simulink model "Md61Md62CalibSet"  (R2018b)
settings: Solver=FixedStepDiscrete  StartTime=0.0  StopTime=10.0  FixedStep=0.01  RelTol=1e-3
undefined symbols (not defined in the file or in its folder): KeSMSuFirstRwStBackPosDelta_Val, KeSMSuFirstRwStCushFoldPosDelta_Val, KeSMSuFirstRwStFwdBkwdPosDelta_Val, KeSMSuThrdRwCushFoldPosDelta_Val, KeSMSwAcsMd30PassStBkReclnUpwdDnwdPos1_Val, KeSMSwAcsMd30PassStBkReclnUpwdDnwdPos1Max_Val, KeSMSwAcsMd30PassStBkReclnUpwdDnwdPos1Min_Val, KeSMSwAcsMd30PassStFldUpwdDnwdPos1_Val, KeSMSwAcsMd30PassStFrwdBkwdPos1_Val, KeSMSwAcsMd30PassStFrwdBkwdPos1Max_Val, KeSMSwAcsMd30PassStFrwdBkwdPos1Min_Val, KeSMSwSeatBkLimitPos_Val, KeSMSwSeatBkLimitPosDelt_Val
libraries: StIsPosChkLib x2
(part 4 of 5)

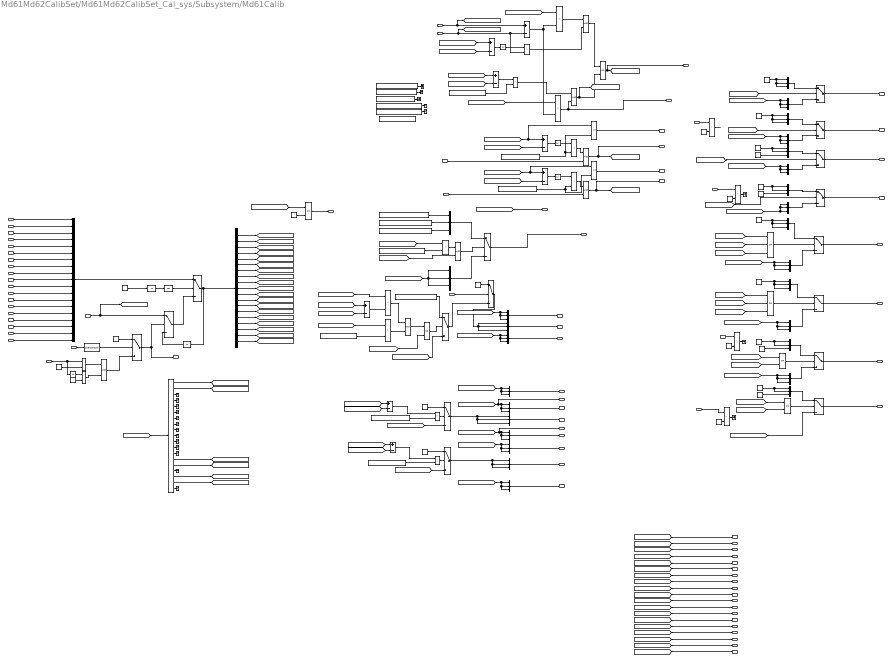
== system Md61Md62CalibSet/Md61Md62CalibSet_Cal_sys/Subsystem/Md61Calib ==
  EepMd61PassStBkReclnTrgtPos_Val_read : Inport
  EepMd61PassStCshnFldTrgtPos_Val_read : Inport  Port=2
  EepMd61PassStFwdBkwdTrgtPos_Val_read : Inport  Port=3
  EepMd61SecRwLtStBkReclnTrgtPos_Val_read : Inport  Port=4
  EepMd61SecRwLtStCushFrntTrgtPos_Val_read : Inport  Port=5
  EepMd61SecRwLtStFwdBkwdTrgtPos_Val_read : Inport  Port=6
  EepMd61SecRwLtStLgrstInwdOtwdTrgtPos_Val_read : Inport  Port=7
  EepMd61SecRwLtStLgrstUpwdDnwdTrgtPos_Val_read : Inport  Port=8
  EepMd61SecRwRtStBkReclnTrgtPos_Val_read : Inport  Port=9
  EepMd61SecRwRtStCushFrntTrgtPos_Val_read : Inport  Port=10
  EepMd61SecRwRtStFwdBkwdTrgtPos_Val_read : Inport  Port=11
  EepMd61SecRwRtStLgrstInwdOtwdTrgtPos_Val_read : Inport  Port=12
  EepMd61SecRwRtStLgrstUpwdDnwdTrgtPos_Val_read : Inport  Port=13
  EepMd61ThdRwLtStBkReclnTrgtPos_Val_read : Inport  Port=14
  EepMd61ThdRwLtStCshnFldTrgtPos_Val_read : Inport  Port=15
  EepMd61ThdRwLtStFwdBkwdTrgtPos_Val_read : Inport  Port=16
  EepMd61ThdRwRtStBkReclnTrgtPos_Val_read : Inport  Port=17
  EepMd61ThdRwRtStCshnFldTrgtPos_Val_read : Inport  Port=18
  EepMd61ThdRwRtStFwdBkwdTrgtPos_Val_read : Inport  Port=19
  CurrentPosArray : Inport  Port=20
  MemReq : Inport  Port=21
  ThdRwLtStCshnFldUpwdDnwdMovConfig : Inport  Port=22
  ThdRwRtStCshnFldUpwdDnwdMovConfig : Inport  Port=23
  KeSMSwSeatBkLimitPos_Val : Inport  Port=24
  KeSMSwSeatBkLimitPosDelt_Val : Inport  Port=25
  IfVeSMSuPassStBkReclnUpwdDnwdPosV_Val_read : Inport  Port=26
  IfVeSMSuSecRwRtStBkReclnUpwdDnwdPos : Inport  Port=27
  IfVeSMSuSecRwLtStFrwdBkwdPos : Inport  Port=28
  IfVeSMSuSecRwLtStBkReclnUpwdDnwdPos : Inport  Port=29
  IfVeSMSuSecRwRtStFrwdBkwdPos : Inport  Port=30
  modestate32_Val_read : Inport  Port=31
  32BitSelector1 : StIsPosChkLib/32BitSelector  BitNum=5
  Abs : Abs
  Abs1 : Abs
  Abs2 : Abs
  Add{,1..3,6..7} (6 alike) : Sum  Inputs=+-  OutDataTypeStr=int16
  Add4 : Sum  Inputs=+-  AccumDataTypeStr=int16  OutDataTypeStr=int16
  Add5 : Sum  Inputs=+-  AccumDataTypeStr=int16  OutDataTypeStr=int16
  Constant : Constant  Value=0  OutDataTypeStr=boolean
  Constant1 : Constant  Value=4  OutDataTypeStr=uint8
  Constant{5..6,9..11,14,26..27} (8 alike) : Constant  Value=0  OutDataTypeStr=uint16
  Constant{7,12,22,24} (4 alike) : Constant  Value=1280  OutDataTypeStr=uint16
  Constant{8,13,23,25} (4 alike) : Constant  Value=480  OutDataTypeStr=uint16
  Constant16 : Constant  Value=4000  OutDataTypeStr=uint16
  Constant18 : Constant  Value=4000  OutDataTypeStr=uint16
  Constant2 : Constant  Value=4  OutDataTypeStr=uint8
  Constant20 : Constant  Value=4095  OutDataTypeStr=uint16
  Constant3 : Constant  Value=0  OutDataTypeStr=uint8
  Constant4 : Constant  Value=4095
  Demux : Demux  Outputs=19
  Demux1 : Demux  Outputs=19
  Logical Operator{,1..3,5,10..11} (7 alike) : Logic  AllPortsSameDT=off  OutDataTypeStr=boolean
  Logical Operator{4,8..9,12} (4 alike) : Logic  Operator=OR  AllPortsSameDT=off  OutDataTypeStr=boolean
  Logical Operator6 : Logic  Operator=OR  Inputs=3  AllPortsSameDT=off  OutDataTypeStr=boolean
  Logical Operator7 : Logic  Operator=OR  Inputs=3  AllPortsSameDT=off  OutDataTypeStr=boolean
  Mux : Mux  Inputs=19
  Mux{2..28} (27 alike) : Mux  Inputs=3
  PA_KeSMSuFirstRwStBackPosDelta_Val : Constant  Value=KeSMSuFirstRwStBackPosDelta_Val
  PA_KeSMSuFirstRwStBackPosDelta_Val1 : Constant  Value=KeSMSuFirstRwStBackPosDelta_Val
  PA_KeSMSuFirstRwStBackPosDelta_Val2 : Constant  Value=KeSMSuFirstRwStBackPosDelta_Val
  PA_KeSMSuFirstRwStCushFoldPosDelta_Val : Constant  Value=KeSMSuFirstRwStCushFoldPosDelta_Val
  PA_KeSMSuFirstRwStFwdBkwdPosDelta_Val : Constant  Value=KeSMSuFirstRwStFwdBkwdPosDelta_Val
  PA_KeSMSuThrdRwCushFoldPosDelta_Val{,1..4} (5 alike) : Constant  Value=KeSMSuThrdRwCushFoldPosDelta_Val
  PA_KeSMSwAcsMd30PassStBkReclnUpwdDnwdPos1Max_Val1 : Constant  Value=KeSMSwAcsMd30PassStBkReclnUpwdDnwdPos1Max_Val
  PA_KeSMSwAcsMd30PassStBkReclnUpwdDnwdPos1Min_Val1 : Constant  Value=KeSMSwAcsMd30PassStBkReclnUpwdDnwdPos1Min_Val
  PA_KeSMSwAcsMd30PassStBkReclnUpwdDnwdPos1_Val1 : Constant  Value=KeSMSwAcsMd30PassStBkReclnUpwdDnwdPos1_Val
  PA_KeSMSwAcsMd30PassStFldUpwdDnwdPos1_Val : Constant  Value=KeSMSwAcsMd30PassStFldUpwdDnwdPos1_Val
  PA_KeSMSwAcsMd30PassStFrwdBkwdPos1Max_Val : Constant  Value=KeSMSwAcsMd30PassStFrwdBkwdPos1Max_Val
  PA_KeSMSwAcsMd30PassStFrwdBkwdPos1Min_Val : Constant  Value=KeSMSwAcsMd30PassStFrwdBkwdPos1Min_Val
  PA_KeSMSwAcsMd30PassStFrwdBkwdPos1_Val : Constant  Value=KeSMSwAcsMd30PassStFrwdBkwdPos1_Val
  Relational Operator : RelationalOperator  Operator===  OutDataTypeStr=boolean  RndMeth=Simplest
  Relational Operator1 : RelationalOperator  Operator=~=  OutDataTypeStr=boolean  RndMeth=Simplest
  Relational Operator10 : RelationalOperator  Operator=<=  OutDataTypeStr=boolean  RndMeth=Simplest
  Relational Operator{2..3,8,11..12,14..20} (12 alike) : RelationalOperator  Operator=>  OutDataTypeStr=boolean  RndMeth=Simplest
  Relational Operator13 : RelationalOperator  Operator=<  OutDataTypeStr=boolean  RndMeth=Simplest
  Relational Operator4 : RelationalOperator  Operator=<  OutDataTypeStr=boolean  RndMeth=Simplest
  Relational Operator6 : RelationalOperator  Operator=<  OutDataTypeStr=boolean  RndMeth=Simplest
  Relational Operator7 : RelationalOperator  Operator===  OutDataTypeStr=boolean  RndMeth=Simplest
  Relational Operator9 : RelationalOperator  Operator=<=  OutDataTypeStr=boolean  RndMeth=Simplest
  Switch{,1..15} (16 alike) : Switch  Criteria=u2 > Threshold
  Terminator_{2..22} (21 alike) : Terminator
  Unit Delay : UnitDelay  InitialCondition=1  SampleTime=-1
  Unit Delay1 : UnitDelay  InitialCondition=1  SampleTime=-1
  Unit Delay2 : UnitDelay  InitialCondition=1  SampleTime=-1
  Unit Delay3 : UnitDelay  SampleTime=-1
  Md61PassStBkReclnTrgtPos_Val_write : Outport
      settings: EnsureOutportIsVirtual=on
  Md61PassStBkReclnTrgtPosCalib_TrgtPosArray_write : Outport  Port=2
      settings: EnsureOutportIsVirtual=on
  Md61PassStCshnFldTrgtPosCalib_TrgtPosArray_write : Outport  Port=3
      settings: EnsureOutportIsVirtual=on
  Md61PassStFwdBkwdTrgtPosCalib_TrgtPosArray_write : Outport  Port=4
      settings: EnsureOutportIsVirtual=on
  Md61SecRwLtStBkReclnTrgtPosCalib_TrgtPosArray_write : Outport  Port=5
      settings: EnsureOutportIsVirtual=on
  Md61SecRwLtStCushFrntTrgtPosCalib_TrgtPosArray_write : Outport  Port=6
      settings: EnsureOutportIsVirtual=on
  Md61SecRwLtStFwdBkwdCalib_TrgtPosArray_write : Outport  Port=7
      settings: EnsureOutportIsVirtual=on
  Md61SecRwLtStLgrstInwdOtwdTrgtPosCalib_TrgtPosArray_write : Outport  Port=8
      settings: EnsureOutportIsVirtual=on
  Md61SecRwLtStLgrstUpwdDnwdTrgtPosCalib_TrgtPosArray_write : Outport  Port=9
      settings: EnsureOutportIsVirtual=on
  Md61ThdRwLtStBkReclnUpwdDnwdTrgtPosCalib_TrgtPosArray_write : Outport  Port=10
      settings: EnsureOutportIsVirtual=on
  Md61ThdRwLtStCshnFldUpwdDnwdTrgtPos_Val_write : Outport  Port=11
      settings: EnsureOutportIsVirtual=on
  Md61ThdRwLtStCshnFldUpwdDnwdTrgtPosCalib_TrgtPosArray_write : Outport  Port=12
      settings: EnsureOutportIsVirtual=on
  Md61ThdRwLtStFrwdBkwdPosTrgtPosCalib_TrgtPosArray_write : Outport  Port=13
      settings: EnsureOutportIsVirtual=on
  Md61ThdRwRtStCshnFldUpwdDnwdTrgtPos_Val_write : Outport  Port=14
      settings: EnsureOutportIsVirtual=on
  Md61SecRwRtStBkReclnTrgtPosCalib_TrgtPosArray_write : Outport  Port=15
      settings: EnsureOutportIsVirtual=on
  Md61SecRwRtStCushFrntTrgtPosCalib_TrgtPosArray_write : Outport  Port=16
      settings: EnsureOutportIsVirtual=on
  Md61SecRwRtStFwdBkwdCalib_TrgtPosArray_write : Outport  Port=17
      settings: EnsureOutportIsVirtual=on
  Md61SecRwRtStLgrstInwdOtwdTrgtPosCalib_TrgtPosArray_write : Outport  Port=18
      settings: EnsureOutportIsVirtual=on
  Md61SecRwRtStLgrstUpwdDnwdTrgtPosCalib_TrgtPosArray_write : Outport  Port=19
      settings: EnsureOutportIsVirtual=on
  Md61ThdRwRtStBkReclnUpwdDnwdTrgtPosCalib_TrgtPosArray_write : Outport  Port=20
      settings: EnsureOutportIsVirtual=on
  Md61ThdRwRtStCshnFldUpwdDnwdTrgtPosCalib_TrgtPosArray_write : Outport  Port=21
      settings: EnsureOutportIsVirtual=on
  Md61ThdRwRtStFrwdBkwdPosTrgtPosCalib_TrgtPosArray_write : Outport  Port=22
      settings: EnsureOutportIsVirtual=on
  Md61PassStNeedFldOpn_Val_write : Outport  Port=23
      settings: EnsureOutportIsVirtual=on
  Md61PassStTrgtIsFld_Val_write : Outport  Port=24
      settings: EnsureOutportIsVirtual=on
  Md61ThdRwLtStNeedFldOpn_Val_write : Outport  Port=25
      settings: EnsureOutportIsVirtual=on
  Md61ThdRwLtStTrgtIsFld_Val_write : Outport  Port=26
      settings: EnsureOutportIsVirtual=on
  Md61ThdRwRtStNeedFldOpn_Val_write : Outport  Port=27
      settings: EnsureOutportIsVirtual=on
  Md61ThdRwRtStTrgtIsFld_Val_write : Outport  Port=28
      settings: EnsureOutportIsVirtual=on
  EepMd61PassStBkReclnTrgtPos_S_Val_write : Outport  Port=29
      settings: EnsureOutportIsVirtual=on
  EepMd61PassStCshnFldTrgtPos_S_Val_write : Outport  Port=30
      settings: EnsureOutportIsVirtual=on
  EepMd61PassStFwdBkwdTrgtPos_S_Val_write : Outport  Port=31
      settings: EnsureOutportIsVirtual=on
  EepMd61SecRwLtStBkReclnTrgtPos_S_Val_write : Outport  Port=32
      settings: EnsureOutportIsVirtual=on
  EepMd61SecRwLtStCushFrntTrgtPos_S_Val_write : Outport  Port=33
      settings: EnsureOutportIsVirtual=on
  EepMd61SecRwLtStFwdBkwdTrgtPos_S_Val_write : Outport  Port=34
      settings: EnsureOutportIsVirtual=on
  EepMd61SecRwLtStLgrstInwdOtwdTrgtPos_S_Val_write : Outport  Port=35
      settings: EnsureOutportIsVirtual=on
  EepMd61SecRwLtStLgrstUpwdDnwdTrgtPos_S_Val_write : Outport  Port=36
      settings: EnsureOutportIsVirtual=on
  EepMd61SecRwRtStBkReclnTrgtPos_S_Val_write : Outport  Port=37
      settings: EnsureOutportIsVirtual=on
  EepMd61SecRwRtStCushFrntTrgtPos_S_Val_write : Outport  Port=38
      settings: EnsureOutportIsVirtual=on
  EepMd61SecRwRtStFwdBkwdTrgtPos_S_Val_write : Outport  Port=39
      settings: EnsureOutportIsVirtual=on
  EepMd61SecRwRtStLgrstInwdOtwdTrgtPos_S_Val_write : Outport  Port=40
      settings: EnsureOutportIsVirtual=on
  EepMd61SecRwRtStLgrstUpwdDnwdTrgtPos_S_Val_write : Outport  Port=41
      settings: EnsureOutportIsVirtual=on
  EepMd61ThdRwLtStBkReclnTrgtPos_S_Val_write : Outport  Port=42
      settings: EnsureOutportIsVirtual=on
  EepMd61ThdRwLtStCshnFldTrgtPos_S_Val_write : Outport  Port=43
      settings: EnsureOutportIsVirtual=on
  EepMd61ThdRwLtStFwdBkwdTrgtPos_S_Val_write : Outport  Port=44
      settings: EnsureOutportIsVirtual=on
  EepMd61ThdRwRtStBkReclnTrgtPos_S_Val_write : Outport  Port=45
      settings: EnsureOutportIsVirtual=on
  EepMd61ThdRwRtStCshnFldTrgtPos_S_Val_write : Outport  Port=46
      settings: EnsureOutportIsVirtual=on
  EepMd61ThdRwRtStFwdBkwdTrgtPos_S_Val_write : Outport  Port=47
      settings: EnsureOutportIsVirtual=on
  Md61MemReq_Val_write : Outport  Port=48
      settings: EnsureOutportIsVirtual=on
  Md61NotMem_Val_write : Outport  Port=49
      settings: EnsureOutportIsVirtual=on
  wires:
  Unit Delay/1 -> Unit Delay1/1
  Constant/1 -> Unit Delay/1
  Unit Delay1/1 -> Switch/2
  Switch1/1 -> Switch/3
  EepMd61ThdRwRtStFwdBkwdTrgtPos_Val_read/1 -> Mux/19
  EepMd61ThdRwRtStCshnFldTrgtPos_Val_read/1 -> Mux/18
  EepMd61ThdRwRtStBkReclnTrgtPos_Val_read/1 -> Mux/17
  EepMd61ThdRwLtStFwdBkwdTrgtPos_Val_read/1 -> Mux/16
  EepMd61ThdRwLtStCshnFldTrgtPos_Val_read/1 -> Mux/15
  EepMd61ThdRwLtStBkReclnTrgtPos_Val_read/1 -> Mux/14
  EepMd61SecRwRtStLgrstUpwdDnwdTrgtPos_Val_read/1 -> Mux/13
  EepMd61SecRwRtStLgrstInwdOtwdTrgtPos_Val_read/1 -> Mux/12
  EepMd61SecRwRtStFwdBkwdTrgtPos_Val_read/1 -> Mux/11
  EepMd61SecRwRtStCushFrntTrgtPos_Val_read/1 -> Mux/10
  EepMd61SecRwRtStBkReclnTrgtPos_Val_read/1 -> Mux/9
  EepMd61SecRwLtStLgrstUpwdDnwdTrgtPos_Val_read/1 -> Mux/8
  EepMd61SecRwLtStLgrstInwdOtwdTrgtPos_Val_read/1 -> Mux/7
  EepMd61SecRwLtStFwdBkwdTrgtPos_Val_read/1 -> Mux/6
  EepMd61SecRwLtStCushFrntTrgtPos_Val_read/1 -> Mux/5
  EepMd61SecRwLtStBkReclnTrgtPos_Val_read/1 -> Mux/4
  EepMd61PassStFwdBkwdTrgtPos_Val_read/1 -> Mux/3
  EepMd61PassStCshnFldTrgtPos_Val_read/1 -> Mux/2
  EepMd61PassStBkReclnTrgtPos_Val_read/1 -> Mux/1
  Mux/1 -> Switch/1
  CurrentPosArray/1 -> [CurrentPosArray], Switch1/1
  Unit Delay2/1 -> Switch1/3
  MemReq/1 -> Unit Delay3/1, Relational Operator/1
  Constant1/1 -> Relational Operator/2
  Relational Operator/1 -> Logical Operator/1
  Unit Delay3/1 -> Relational Operator1/1
  Constant2/1 -> Relational Operator1/2
  Relational Operator1/1 -> Logical Operator/2
  Demux/15 -> [ThdRwLtStCshnFldTrgtPos]
  Demux/16 -> [ThdRwLtStFwdBkwdTrgtPos]
  Demux/5 -> [SecRwLtStCushFrntTrgtPos]
  Demux/17 -> [ThdRwRtStBkReclnTrgtPos]
  Demux/14 -> [ThdRwLtStBkReclnTrgtPos]
  Demux/9 -> [SecRwRtStBkReclnTrgtPos]
  Demux/13 -> [SecRwRtStLgrstUpwdDnwdTrgtPos]
  Demux/19 -> [ThdRwRtStFwdBkwdTrgtPos]
  Demux/11 -> [SecRwRtStFwdBkwdTrgtPos]
  Switch/1 -> Demux/1, Unit Delay2/1
  Demux/8 -> [SecRwLtStLgrstUpwdDnwdTrgtPos]
  Demux/2 -> [PassStCshnFldTrgtPos]
  Demux/12 -> [SecRwRtStLgrstInwdOtwdTrgtPos]
  Demux/7 -> [SecRwLtStLgrstInwdOtwdTrgtPos]
  Demux/6 -> [SecRwLtStFwdBkwdTrgtPos]
  Demux/4 -> [SecRwLtStBkReclnTrgtPos]
  Demux/3 -> [PassStFwdBkwdTrgtPos]
  Demux/1 -> [PassStBkReclnTrgtPos]
  Demux/10 -> [SecRwRtStCushFrntTrgtPos]
  Demux/18 -> [ThdRwRtStCshnFldTrgtPos]
  Mux2/1 -> Md61PassStCshnFldTrgtPosCalib_TrgtPosArray_write/1
  [PassStCshnFldTrgtPos] -> Mux2/1, Mux2/2, Mux2/3
  Mux3/1 -> Md61PassStFwdBkwdTrgtPosCalib_TrgtPosArray_write/1
  Mux4/1 -> Md61SecRwLtStCushFrntTrgtPosCalib_TrgtPosArray_write/1
  [SecRwLtStCushFrntTrgtPos] -> Mux4/1, Mux4/2, Mux4/3
  [ThdRwLtStBkReclnTrgtPos] -> Mux5/3, Mux5/2, Mux5/1
  Mux5/1 -> Md61ThdRwLtStBkReclnUpwdDnwdTrgtPosCalib_TrgtPosArray_write/1
  [ThdRwLtStCshnFldTrgtPos] -> Md61ThdRwLtStCshnFldUpwdDnwdTrgtPos_Val_write/1, Mux6/1, Mux6/2, Mux6/3
  Mux6/1 -> Md61ThdRwLtStCshnFldUpwdDnwdTrgtPosCalib_TrgtPosArray_write/1
  Mux7/1 -> Md61ThdRwLtStFrwdBkwdPosTrgtPosCalib_TrgtPosArray_write/1
  [ThdRwRtStCshnFldTrgtPos] -> Md61ThdRwRtStCshnFldUpwdDnwdTrgtPos_Val_write/1, Mux8/1, Mux8/2, Mux8/3
  [SecRwRtStCushFrntTrgtPos] -> Mux9/3, Mux9/2, Mux9/1
  Mux9/1 -> Md61SecRwRtStCushFrntTrgtPosCalib_TrgtPosArray_write/1
  Mux8/1 -> Md61ThdRwRtStCshnFldUpwdDnwdTrgtPosCalib_TrgtPosArray_write/1
  Mux10/1 -> Md61ThdRwRtStBkReclnUpwdDnwdTrgtPosCalib_TrgtPosArray_write/1
  [ThdRwRtStBkReclnTrgtPos] -> Mux10/3, Mux10/2, Mux10/1
  Mux11/1 -> Md61ThdRwRtStFrwdBkwdPosTrgtPosCalib_TrgtPosArray_write/1
  [CurrentPosArray] -> Demux1/1
  Demux1/17 -> [ThdRwRtStBkReclnPos]
  Demux1/14 -> [ThdRwLtStBkReclnPos]
  Demux1/18 -> [ThdRwRtStCshnFldPos]
  Demux1/1 -> [PassStBkReclnPos]
  Demux1/15 -> [ThdRwLtStCshnFldPos]
  Demux1/2 -> [PassStCshnFldPos]
  [ThdRwLtStCshnFldPos] -> Add/2
  Add/1 -> Abs/1
  Abs/1 -> Relational Operator2/1
  PA_KeSMSuThrdRwCushFoldPosDelta_Val1/1 -> Relational Operator9/2, Relational Operator2/2
  ThdRwLtStCshnFldUpwdDnwdMovConfig/1 -> Logical Operator1/2
  Relational Operator2/1 -> Logical Operator1/1
  Logical Operator1/1 -> Md61ThdRwLtStNeedFldOpn_Val_write/1, [ThdLftNeedFldOpn]
  ThdRwRtStCshnFldUpwdDnwdMovConfig/1 -> Logical Operator2/2
  Relational Operator3/1 -> Logical Operator2/1
  PA_KeSMSuThrdRwCushFoldPosDelta_Val2/1 -> Relational Operator3/2, Relational Operator10/2
  Abs1/1 -> Relational Operator3/1
  Add1/1 -> Abs1/1
  [ThdRwRtStCshnFldPos] -> Add1/2
  [ThdRwRtStCshnFldTrgtPos] -> Relational Operator10/1, Add1/1
  Logical Operator2/1 -> Md61ThdRwRtStNeedFldOpn_Val_write/1, [ThdRghtNeedFldOpn]
  Demux1/3 -> Terminator_2/1
  Demux1/4 -> Terminator_3/1
  Demux1/5 -> Terminator_4/1
  Demux1/6 -> Terminator_5/1
  Demux1/7 -> Terminator_6/1
  Demux1/8 -> Terminator_7/1
  Demux1/9 -> Terminator_8/1
  Demux1/10 -> Terminator_9/1
  Demux1/11 -> Terminator_10/1
  Demux1/12 -> Terminator_11/1
  Demux1/13 -> Terminator_12/1
  Demux1/16 -> Terminator_13/1
  Demux1/19 -> Terminator_14/1
  [ThdLftNeedFldOpn] -> Switch2/2
  Switch8/1 -> Md61SecRwRtStBkReclnTrgtPosCalib_TrgtPosArray_write/1
  KeSMSwSeatBkLimitPosDelt_Val/1 -> [SeatBkLimitPosDelt], Relational Operator8/2, Add2/2
  [PassStBkReclnPos] -> Relational Operator4/1
  Relational Operator4/1 -> Logical Operator3/1
  Logical Operator3/1 -> Logical Operator4/1
  Logical Operator4/1 -> Md61PassStNeedFldOpn_Val_write/1, [PassStNeedFldOpn]
  KeSMSwSeatBkLimitPos_Val/1 -> [SeatBkLimitPos], Add2/1
  Logical Operator5/1 -> [PassStNeedFld], Logical Operator4/2
  Relational Operator6/1 -> Md61PassStTrgtIsFld_Val_write/1, Logical Operator5/2
  Add2/1 -> Relational Operator6/2, Relational Operator4/2
  [PassStBkReclnTrgtPos] -> Relational Operator6/1
  [PassStBkReclnPos] -> Add3/2
  [PassStBkReclnTrgtPos] -> Add3/1
  Add3/1 -> Abs2/1
  Abs2/1 -> Relational Operator8/1
  Relational Operator8/1 -> Logical Operator3/2
  [ThdLftNeedFldOpn] -> Logical Operator6/1
  [ThdRghtNeedFldOpn] -> Logical Operator6/2
  Mux12/1 -> Switch2/1
  Switch2/1 -> Md61SecRwLtStLgrstInwdOtwdTrgtPosCalib_TrgtPosArray_write/1
  Switch3/1 -> Md61SecRwLtStLgrstUpwdDnwdTrgtPosCalib_TrgtPosArray_write/1
  [ThdLftNeedFldOpn] -> Switch3/2
  [SecRwLtStLgrstInwdOtwdTrgtPos] -> Mux13/1, Mux13/2, Mux13/3
  Mux13/1 -> Switch2/3
  Mux14/1 -> Switch3/3
  [SecRwLtStLgrstUpwdDnwdTrgtPos] -> Mux14/3, Mux14/2, Mux14/1
  Constant5/1 -> Mux12/3, Mux12/2, Mux12/1
  Constant6/1 -> Mux15/3, Mux15/2, Mux15/1
  Mux15/1 -> Switch3/1
  Switch4/1 -> Md61SecRwLtStBkReclnTrgtPosCalib_TrgtPosArray_write/1
  Switch5/1 -> Md61SecRwLtStFwdBkwdCalib_TrgtPosArray_write/1
  [SecRwLtStBkReclnTrgtPos] -> Mux16/1, Mux16/2, Mux16/3
  Mux16/1 -> Switch4/3
  Mux17/1 -> Switch5/3
  [SecRwLtStFwdBkwdTrgtPos] -> Mux17/1, Mux17/2, Mux17/3
  Mux18/1 -> Switch4/1
  Constant7/1 -> Mux18/1, Mux18/2
  Constant8/1 -> Mux19/2, Mux19/1
  Mux19/1 -> Switch5/1
  Constant9/1 -> Mux19/3
  [PassStNeedFldOpn] -> Logical Operator6/3
  Switch6/1 -> Md61SecRwRtStLgrstInwdOtwdTrgtPosCalib_TrgtPosArray_write/1
  Mux20/1 -> Switch6/1
  Logical Operator6/1 -> Switch6/2
  Logical Operator7/1 -> Switch7/2
  Mux21/1 -> Switch7/1
  Switch7/1 -> Md61SecRwRtStLgrstUpwdDnwdTrgtPosCalib_TrgtPosArray_write/1
  [PassStNeedFldOpn] -> Logical Operator7/3
  [ThdRghtNeedFldOpn] -> Logical Operator7/2
  [ThdLftNeedFldOpn] -> Logical Operator7/1
  Constant10/1 -> Mux20/1, Mux20/2, Mux20/3
  Constant11/1 -> Mux21/3, Mux21/2, Mux21/1
  [SecRwRtStLgrstInwdOtwdTrgtPos] -> Mux22/3, Mux22/2, Mux22/1
  Mux22/1 -> Switch6/3
  Mux23/1 -> Switch7/3
  [SecRwRtStLgrstUpwdDnwdTrgtPos] -> Mux23/3, Mux23/2, Mux23/1
  Switch9/1 -> Md61SecRwRtStFwdBkwdCalib_TrgtPosArray_write/1
  Mux24/1 -> Switch8/1
  [ThdLftNeedFldOpn] -> Logical Operator8/1
  [ThdRghtNeedFldOpn] -> Logical Operator8/2
  Constant12/1 -> Mux24/2, Mux24/1
  [SecRwRtStBkReclnTrgtPos] -> Mux25/1, Mux25/2, Mux25/3
  Mux25/1 -> Switch8/3
  Constant14/1 -> Mux26/3
  Mux26/1 -> Switch9/1
  Constant13/1 -> Mux26/1, Mux26/2
  [ThdRghtNeedFldOpn] -> Logical Operator9/2
  [ThdLftNeedFldOpn] -> Logical Operator9/1
  [SecRwRtStFwdBkwdTrgtPos] -> Switch9/3
  [ThdRwLtStCshnFldTrgtPos] -> Relational Operator9/1, Add/1
  Relational Operator10/1 -> Md61ThdRwRtStTrgtIsFld_Val_write/1
  Relational Operator9/1 -> Md61ThdRwLtStTrgtIsFld_Val_write/1
  [ThdRwLtStFwdBkwdTrgtPos] -> Switch10/3
  Switch10/1 -> Mux7/3, Mux7/2, Mux7/1
  [ThdRwLtStCshnFldTrgtPos] -> Add4/2
  [ThdRwLtStCshnFldPos] -> Add4/1
  Add4/1 -> Relational Operator11/1
  PA_KeSMSuThrdRwCushFoldPosDelta_Val3/1 -> Relational Operator11/2
  Relational Operator11/1 -> Switch10/2
  Constant16/1 -> Switch10/1
  Switch11/1 -> Mux11/3, Mux11/2, Mux11/1
  [ThdRwRtStFwdBkwdTrgtPos] -> Switch11/3
  Constant18/1 -> Switch11/1
  Add5/1 -> Relational Operator12/1
  Relational Operator12/1 -> Switch11/2
  [ThdRwRtStCshnFldTrgtPos] -> Add5/2
  PA_KeSMSuThrdRwCushFoldPosDelta_Val4/1 -> Relational Operator12/2
  [ThdRwRtStCshnFldPos] -> Add5/1
  [SeatBkLimitPos] -> Add6/1
  [SeatBkLimitPosDelt] -> Add6/2
  [PassStBkReclnPos] -> Relational Operator13/1
  Add6/1 -> Relational Operator13/2
  PA_KeSMSuFirstRwStBackPosDelta_Val1/1 -> Relational Operator14/2
  [PassStBkReclnPos] -> Relational Operator14/1
  Relational Operator13/1 -> Logical Operator10/1
  Relational Operator14/1 -> Logical Operator10/2
  [PassStFwdBkwdTrgtPos] -> Switch12/3
  Switch15/1 -> Mux3/2, Mux3/3, Mux3/1
  PA_KeSMSwAcsMd30PassStFrwdBkwdPos1_Val/1 -> Switch12/1
  PA_KeSMSwAcsMd30PassStFldUpwdDnwdPos1_Val/1 -> Relational Operator15/2
  [PassStCshnFldPos] -> Relational Operator15/1
  PA_KeSMSwAcsMd30PassStBkReclnUpwdDnwdPos1_Val1/1 -> Mux27/1
  PA_KeSMSwAcsMd30PassStBkReclnUpwdDnwdPos1Max_Val1/1 -> Mux27/2
  Mux27/1 -> Switch13/1
  [PassStBkReclnTrgtPos] -> Md61PassStBkReclnTrgtPos_Val_write/1
  [PassStBkReclnTrgtPos] -> Mux28/3, Mux28/1, Mux28/2
  Mux28/1 -> Switch13/3
  Switch13/1 -> Md61PassStBkReclnTrgtPosCalib_TrgtPosArray_write/1
  Relational Operator15/1 -> Logical Operator11/1
  Logical Operator11/1 -> Switch13/2
  [PassStBkReclnPos] -> Add7/1
  [PassStBkReclnTrgtPos] -> Add7/2
  Add7/1 -> Relational Operator16/1
  PA_KeSMSuFirstRwStBackPosDelta_Val/1 -> Relational Operator16/2
  Relational Operator16/1 -> Logical Operator5/1
  [PassStNeedFld] -> Logical Operator11/2
  PA_KeSMSwAcsMd30PassStBkReclnUpwdDnwdPos1Min_Val1/1 -> Mux27/3
  [PassStBkReclnTrgtPos] -> EepMd61PassStBkReclnTrgtPos_S_Val_write/1
  [PassStCshnFldTrgtPos] -> EepMd61PassStCshnFldTrgtPos_S_Val_write/1
  [PassStFwdBkwdTrgtPos] -> EepMd61PassStFwdBkwdTrgtPos_S_Val_write/1
  [SecRwLtStBkReclnTrgtPos] -> EepMd61SecRwLtStBkReclnTrgtPos_S_Val_write/1
  [SecRwLtStCushFrntTrgtPos] -> EepMd61SecRwLtStCushFrntTrgtPos_S_Val_write/1
  [ThdRwRtStFwdBkwdTrgtPos] -> EepMd61ThdRwRtStFwdBkwdTrgtPos_S_Val_write/1
  [ThdRwRtStCshnFldTrgtPos] -> EepMd61ThdRwRtStCshnFldTrgtPos_S_Val_write/1
  [ThdRwRtStBkReclnTrgtPos] -> EepMd61ThdRwRtStBkReclnTrgtPos_S_Val_write/1
  [ThdRwLtStFwdBkwdTrgtPos] -> EepMd61ThdRwLtStFwdBkwdTrgtPos_S_Val_write/1
  [ThdRwLtStCshnFldTrgtPos] -> EepMd61ThdRwLtStCshnFldTrgtPos_S_Val_write/1
  [ThdRwLtStBkReclnTrgtPos] -> EepMd61ThdRwLtStBkReclnTrgtPos_S_Val_write/1
  [SecRwRtStLgrstUpwdDnwdTrgtPos] -> EepMd61SecRwRtStLgrstUpwdDnwdTrgtPos_S_Val_write/1
  [SecRwRtStLgrstInwdOtwdTrgtPos] -> EepMd61SecRwRtStLgrstInwdOtwdTrgtPos_S_Val_write/1
  [SecRwRtStFwdBkwdTrgtPos] -> EepMd61SecRwRtStFwdBkwdTrgtPos_S_Val_write/1
  [SecRwRtStCushFrntTrgtPos] -> EepMd61SecRwRtStCushFrntTrgtPos_S_Val_write/1
  [SecRwRtStBkReclnTrgtPos] -> EepMd61SecRwRtStBkReclnTrgtPos_S_Val_write/1
  [SecRwLtStLgrstUpwdDnwdTrgtPos] -> EepMd61SecRwLtStLgrstUpwdDnwdTrgtPos_S_Val_write/1
  [SecRwLtStLgrstInwdOtwdTrgtPos] -> EepMd61SecRwLtStLgrstInwdOtwdTrgtPos_S_Val_write/1
  [SecRwLtStFwdBkwdTrgtPos] -> EepMd61SecRwLtStFwdBkwdTrgtPos_S_Val_write/1
  Relational Operator7/1 -> Md61NotMem_Val_write/1
  Constant20/1 -> Relational Operator7/2
  [PassStBkReclnTrgtPos] -> Relational Operator7/1
  Logical Operator12/1 -> Switch12/2
  Logical Operator10/1 -> Logical Operator12/1
  [PassStNeedFldOpn] -> Logical Operator12/2
  Constant22/1 -> Relational Operator17/2
  Relational Operator17/1 -> ?
  [ThdLftNeedFldOpn] -> Switch4/2
  IfVeSMSuSecRwLtStBkReclnUpwdDnwdPos/1 -> Relational Operator17/1
  Constant23/1 -> Relational Operator18/2
  IfVeSMSuSecRwLtStFrwdBkwdPos/1 -> Relational Operator18/1
  [ThdLftNeedFldOpn] -> Switch5/2
  Constant24/1 -> Relational Operator19/2
  Logical Operator8/1 -> Switch8/2
  IfVeSMSuSecRwRtStBkReclnUpwdDnwdPos/1 -> Relational Operator19/1
  Constant25/1 -> Relational Operator20/2
  IfVeSMSuSecRwRtStFrwdBkwdPos/1 -> Relational Operator20/1
  Logical Operator9/1 -> Switch9/2
  Constant26/1 -> Mux24/3
  Constant27/1 -> Mux18/3
  Relational Operator18/1 -> Terminator_15/1
  Relational Operator19/1 -> Terminator_16/1
  Relational Operator20/1 -> Terminator_17/1
  PA_KeSMSwAcsMd30PassStFrwdBkwdPos1Min_Val/1 -> Terminator_22/1
  PA_KeSMSuFirstRwStFwdBkwdPosDelta_Val/1 -> Terminator_19/1
  PA_KeSMSwAcsMd30PassStFrwdBkwdPos1Max_Val/1 -> Terminator_21/1
  PA_KeSMSuThrdRwCushFoldPosDelta_Val/1 -> Terminator_20/1
  PA_KeSMSuFirstRwStCushFoldPosDelta_Val/1 -> Terminator_18/1
  modestate32_Val_read/1 -> 32BitSelector1/1
  32BitSelector1/1 -> Switch14/2
  Constant3/1 -> Switch14/1
  Logical Operator/1 -> Switch14/3
  Switch14/1 -> Md61MemReq_Val_write/1, Switch1/2
  IfVeSMSuPassStBkReclnUpwdDnwdPosV_Val_read/1 -> Switch15/2
  Constant4/1 -> Switch15/1
  Switch12/1 -> Switch15/3

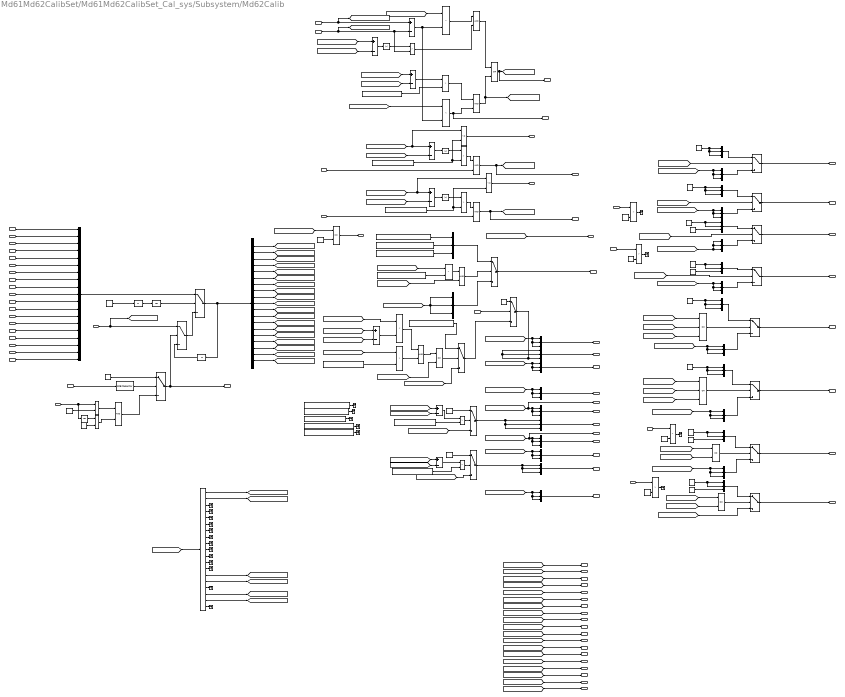
== system Md61Md62CalibSet/Md61Md62CalibSet_Cal_sys/Subsystem/Md62Calib ==
  EepMd62PassStBkReclnTrgtPos_Val_read : Inport
  EepMd62PassStCshnFldTrgtPos_Val_read : Inport  Port=2
  EepMd62PassStFwdBkwdTrgtPos_Val_read : Inport  Port=3
  EepMd62SecRwLtStBkReclnTrgtPos_Val_read : Inport  Port=4
  EepMd62SecRwLtStCushFrntTrgtPos_Val_read : Inport  Port=5
  EepMd62SecRwLtStFwdBkwdTrgtPos_Val_read : Inport  Port=6
  EepMd62SecRwLtStLgrstInwdOtwdTrgtPos_Val_read : Inport  Port=7
  EepMd62SecRwLtStLgrstUpwdDnwdTrgtPos_Val_read : Inport  Port=8
  EepMd62SecRwRtStBkReclnTrgtPos_Val_read : Inport  Port=9
  EepMd62SecRwRtStCushFrntTrgtPos_Val_read : Inport  Port=10
  EepMd62SecRwRtStFwdBkwdTrgtPos_Val_read : Inport  Port=11
  EepMd62SecRwRtStLgrstInwdOtwdTrgtPos_Val_read : Inport  Port=12
  EepMd62SecRwRtStLgrstUpwdDnwdTrgtPos_Val_read : Inport  Port=13
  EepMd62ThdRwLtStBkReclnTrgtPos_Val_read : Inport  Port=14
  EepMd62ThdRwLtStCshnFldTrgtPos_Val_read : Inport  Port=15
  EepMd62ThdRwLtStFwdBkwdTrgtPos_Val_read : Inport  Port=16
  EepMd62ThdRwRtStBkReclnTrgtPos_Val_read : Inport  Port=17
  EepMd62ThdRwRtStCshnFldTrgtPos_Val_read : Inport  Port=18
  EepMd62ThdRwRtStFwdBkwdTrgtPos_Val_read : Inport  Port=19
  CurrentPosArray : Inport  Port=20
  MemReq : Inport  Port=21
  ThdRwLtStCshnFldUpwdDnwdMovConfig : Inport  Port=22
  ThdRwRtStCshnFldUpwdDnwdMovConfig : Inport  Port=23
  KeSMSwSeatBkLimitPos_Val : Inport  Port=24
  KeSMSwSeatBkLimitPosDelt_Val : Inport  Port=25
  IfVeSMSuSecRwRtStBkReclnUpwdDnwdPos : Inport  Port=26
  IfVeSMSuSecRwLtStFrwdBkwdPos : Inport  Port=27
  IfVeSMSuSecRwLtStBkReclnUpwdDnwdPos : Inport  Port=28
  IfVeSMSuSecRwRtStFrwdBkwdPos : Inport  Port=29
  modestate32_Val_read : Inport  Port=30
  IfVeSMSuPassStBkReclnUpwdDnwdPosV : Inport  Port=31
  32BitSelector2 : StIsPosChkLib/32BitSelector  BitNum=6
  Abs : Abs
  Abs1 : Abs
  Abs2 : Abs
  Add{,1..3,6,8} (6 alike) : Sum  Inputs=+-  OutDataTypeStr=int16
  Add4 : Sum  Inputs=+-  AccumDataTypeStr=int16  OutDataTypeStr=int16
  Add5 : Sum  Inputs=+-  AccumDataTypeStr=int16  OutDataTypeStr=int16
  Constant : Constant  Value=0  OutDataTypeStr=boolean
  Constant1 : Constant  Value=5  OutDataTypeStr=uint8
  Constant{3,5..6,9..11,14,26} (8 alike) : Constant  Value=0  OutDataTypeStr=uint16
  Constant12 : Constant  Value=1280  OutDataTypeStr=uint16
  Constant{8,13,22..23,25} (5 alike) : Constant  Value=480  OutDataTypeStr=uint16
  Constant15 : Constant  Value=4095
  Constant16 : Constant  Value=4000  OutDataTypeStr=uint16
  Constant18 : Constant  Value=4000  OutDataTypeStr=uint16
  Constant2 : Constant  Value=5  OutDataTypeStr=uint8
  Constant21 : Constant  Value=4095  OutDataTypeStr=uint16
  Constant24 : Constant  Value=1280  OutDataTypeStr=uint16
  Constant4 : Constant  Value=0  OutDataTypeStr=uint8
  Constant7 : Constant  Value=1280  OutDataTypeStr=uint16
  Demux : Demux  Outputs=19
  Demux1 : Demux  Outputs=19
  Logical Operator{,1..3,5,10..11} (7 alike) : Logic  AllPortsSameDT=off  OutDataTypeStr=boolean
  Logical Operator{4,8..9,12} (4 alike) : Logic  Operator=OR  AllPortsSameDT=off  OutDataTypeStr=boolean
  Logical Operator6 : Logic  Operator=OR  Inputs=3  AllPortsSameDT=off  OutDataTypeStr=boolean
  Logical Operator7 : Logic  Operator=OR  Inputs=3  AllPortsSameDT=off  OutDataTypeStr=boolean
  Mux : Mux  Inputs=19
  Mux{2..28} (27 alike) : Mux  Inputs=3
  PA_KeSMSuFirstRwStBackPosDelta_Val1 : Constant  Value=KeSMSuFirstRwStBackPosDelta_Val
  PA_KeSMSuFirstRwStBackPosDelta_Val2 : Constant  Value=KeSMSuFirstRwStBackPosDelta_Val
  PA_KeSMSuFirstRwStCushFoldPosDelta_Val : Constant  Value=KeSMSuFirstRwStCushFoldPosDelta_Val
  PA_KeSMSuFirstRwStFwdBkwdPosDelta_Val : Constant  Value=KeSMSuFirstRwStFwdBkwdPosDelta_Val
  PA_KeSMSuThrdRwCushFoldPosDelta_Val{,1..4} (5 alike) : Constant  Value=KeSMSuThrdRwCushFoldPosDelta_Val
  PA_KeSMSwAcsMd30PassStBkReclnUpwdDnwdPos1Max_Val1 : Constant  Value=KeSMSwAcsMd30PassStBkReclnUpwdDnwdPos1Max_Val
  PA_KeSMSwAcsMd30PassStBkReclnUpwdDnwdPos1Min_Val1 : Constant  Value=KeSMSwAcsMd30PassStBkReclnUpwdDnwdPos1Min_Val
  PA_KeSMSwAcsMd30PassStBkReclnUpwdDnwdPos1_Val1 : Constant  Value=KeSMSwAcsMd30PassStBkReclnUpwdDnwdPos1_Val
  PA_KeSMSwAcsMd30PassStFldUpwdDnwdPos1_Val : Constant  Value=KeSMSwAcsMd30PassStFldUpwdDnwdPos1_Val
  PA_KeSMSwAcsMd30PassStFrwdBkwdPos1Max_Val : Constant  Value=KeSMSwAcsMd30PassStFrwdBkwdPos1Max_Val
  PA_KeSMSwAcsMd30PassStFrwdBkwdPos1Min_Val : Constant  Value=KeSMSwAcsMd30PassStFrwdBkwdPos1Min_Val
  PA_KeSMSwAcsMd30PassStFrwdBkwdPos1_Val : Constant  Value=KeSMSwAcsMd30PassStFrwdBkwdPos1_Val
  Relational Operator : RelationalOperator  Operator===  OutDataTypeStr=boolean  RndMeth=Simplest
  Relational Operator1 : RelationalOperator  Operator=~=  OutDataTypeStr=boolean  RndMeth=Simplest
  Relational Operator10 : RelationalOperator  Operator=<=  OutDataTypeStr=boolean  RndMeth=Simplest
  Relational Operator{2..3,7..8,11..12,14..15,17..20} (12 alike) : RelationalOperator  Operator=>  OutDataTypeStr=boolean  RndMeth=Simplest
  Relational Operator13 : RelationalOperator  Operator=<  OutDataTypeStr=boolean  RndMeth=Simplest
  Relational Operator16 : RelationalOperator  Operator===  OutDataTypeStr=boolean  RndMeth=Simplest
  Relational Operator4 : RelationalOperator  Operator=<  OutDataTypeStr=boolean  RndMeth=Simplest
  Relational Operator6 : RelationalOperator  Operator=<  OutDataTypeStr=boolean  RndMeth=Simplest
  Relational Operator9 : RelationalOperator  Operator=<=  OutDataTypeStr=boolean  RndMeth=Simplest
  Switch{,1..15} (16 alike) : Switch  Criteria=u2 > Threshold
  Terminator_{1..22} (22 alike) : Terminator
  Unit Delay : UnitDelay  InitialCondition=1  SampleTime=-1
  Unit Delay1 : UnitDelay  InitialCondition=1  SampleTime=-1
  Unit Delay2 : UnitDelay  InitialCondition=1  SampleTime=-1
  Unit Delay3 : UnitDelay  SampleTime=-1
  Md62PassStBkReclnTrgtPos_Val_write : Outport
      settings: EnsureOutportIsVirtual=on
  Md62PassStBkReclnTrgtPosCalib_TrgtPosArray_write : Outport  Port=2
      settings: EnsureOutportIsVirtual=on
  Md62PassStCshnFldTrgtPosCalib_TrgtPosArray_write : Outport  Port=3
      settings: EnsureOutportIsVirtual=on
  Md62PassStFwdBkwdTrgtPosCalib_TrgtPosArray_write : Outport  Port=4
      settings: EnsureOutportIsVirtual=on
  Md62SecRwLtStBkReclnTrgtPosCalib_TrgtPosArray_write : Outport  Port=5
      settings: EnsureOutportIsVirtual=on
  Md62SecRwLtStCushFrntTrgtPosCalib_TrgtPosArray_write : Outport  Port=6
      settings: EnsureOutportIsVirtual=on
  Md62SecRwLtStFwdBkwdCalib_TrgtPosArray_write : Outport  Port=7
      settings: EnsureOutportIsVirtual=on
  Md62SecRwLtStLgrstInwdOtwdTrgtPosCalib_TrgtPosArray_write : Outport  Port=8
      settings: EnsureOutportIsVirtual=on
  Md62SecRwLtStLgrstUpwdDnwdTrgtPosCalib_TrgtPosArray_write : Outport  Port=9
      settings: EnsureOutportIsVirtual=on
  Md62ThdRwLtStBkReclnUpwdDnwdTrgtPosCalib_TrgtPosArray_write : Outport  Port=10
      settings: EnsureOutportIsVirtual=on
  Md62ThdRwLtStCshnFldUpwdDnwdTrgtPos_Val_write : Outport  Port=11
      settings: EnsureOutportIsVirtual=on
  Md62ThdRwLtStCshnFldUpwdDnwdTrgtPosCalib_TrgtPosArray_write : Outport  Port=12
      settings: EnsureOutportIsVirtual=on
  Md62ThdRwLtStFrwdBkwdPosTrgtPosCalib_TrgtPosArray_write : Outport  Port=13
      settings: EnsureOutportIsVirtual=on
  Md62ThdRwRtStCshnFldUpwdDnwdTrgtPos_Val_write : Outport  Port=14
      settings: EnsureOutportIsVirtual=on
  Md62SecRwRtStBkReclnTrgtPosCalib_TrgtPosArray_write : Outport  Port=15
      settings: EnsureOutportIsVirtual=on
  Md62SecRwRtStCushFrntTrgtPosCalib_TrgtPosArray_write : Outport  Port=16
      settings: EnsureOutportIsVirtual=on
  Md62SecRwRtStFwdBkwdCalib_TrgtPosArray_write : Outport  Port=17
      settings: EnsureOutportIsVirtual=on
  Md62SecRwRtStLgrstInwdOtwdTrgtPosCalib_TrgtPosArray_write : Outport  Port=18
      settings: EnsureOutportIsVirtual=on
  Md62SecRwRtStLgrstUpwdDnwdTrgtPosCalib_TrgtPosArray_write : Outport  Port=19
      settings: EnsureOutportIsVirtual=on
  Md62ThdRwRtStBkReclnUpwdDnwdTrgtPosCalib_TrgtPosArray_write : Outport  Port=20
      settings: EnsureOutportIsVirtual=on
  Md62ThdRwRtStCshnFldUpwdDnwdTrgtPosCalib_TrgtPosArray_write : Outport  Port=21
      settings: EnsureOutportIsVirtual=on
  Md62ThdRwRtStFrwdBkwdPosTrgtPosCalib_TrgtPosArray_write : Outport  Port=22
      settings: EnsureOutportIsVirtual=on
  Md62PassStNeedFldOpn_Val_write : Outport  Port=23
      settings: EnsureOutportIsVirtual=on
  Md62PassStTrgtIsFld_Val_write : Outport  Port=24
      settings: EnsureOutportIsVirtual=on
  Md62ThdRwLtStNeedFldOpn_Val_write : Outport  Port=25
      settings: EnsureOutportIsVirtual=on
  Md62ThdRwLtStTrgtIsFld_Val_write : Outport  Port=26
      settings: EnsureOutportIsVirtual=on
  Md62ThdRwRtStNeedFldOpn_Val_write : Outport  Port=27
      settings: EnsureOutportIsVirtual=on
  Md62ThdRwRtStTrgtIsFld_Val_write : Outport  Port=28
      settings: EnsureOutportIsVirtual=on
  EepMd62PassStBkReclnTrgtPos_S_Val_write : Outport  Port=29
      settings: EnsureOutportIsVirtual=on
  EepMd62PassStCshnFldTrgtPos_S_Val_write : Outport  Port=30
      settings: EnsureOutportIsVirtual=on
  EepMd62PassStFwdBkwdTrgtPos_S_Val_write : Outport  Port=31
      settings: EnsureOutportIsVirtual=on
  EepMd62SecRwLtStBkReclnTrgtPos_S_Val_write : Outport  Port=32
      settings: EnsureOutportIsVirtual=on
  EepMd62SecRwLtStCushFrntTrgtPos_S_Val_write : Outport  Port=33
      settings: EnsureOutportIsVirtual=on
  EepMd62SecRwLtStFwdBkwdTrgtPos_S_Val_write : Outport  Port=34
      settings: EnsureOutportIsVirtual=on
  EepMd62SecRwLtStLgrstInwdOtwdTrgtPos_S_Val_write : Outport  Port=35
      settings: EnsureOutportIsVirtual=on
  EepMd62SecRwLtStLgrstUpwdDnwdTrgtPos_S_Val_write : Outport  Port=36
      settings: EnsureOutportIsVirtual=on
  EepMd62SecRwRtStBkReclnTrgtPos_S_Val_write : Outport  Port=37
      settings: EnsureOutportIsVirtual=on
  EepMd62SecRwRtStCushFrntTrgtPos_S_Val_write : Outport  Port=38
      settings: EnsureOutportIsVirtual=on
  EepMd62SecRwRtStFwdBkwdTrgtPos_S_Val_write : Outport  Port=39
      settings: EnsureOutportIsVirtual=on
  EepMd62SecRwRtStLgrstInwdOtwdTrgtPos_S_Val_write : Outport  Port=40
      settings: EnsureOutportIsVirtual=on
  EepMd62SecRwRtStLgrstUpwdDnwdTrgtPos_S_Val_write : Outport  Port=41
      settings: EnsureOutportIsVirtual=on
  EepMd62ThdRwLtStBkReclnTrgtPos_S_Val_write : Outport  Port=42
      settings: EnsureOutportIsVirtual=on
  EepMd62ThdRwLtStCshnFldTrgtPos_S_Val_write : Outport  Port=43
      settings: EnsureOutportIsVirtual=on
  EepMd62ThdRwLtStFwdBkwdTrgtPos_S_Val_write : Outport  Port=44
      settings: EnsureOutportIsVirtual=on
  EepMd62ThdRwRtStBkReclnTrgtPos_S_Val_write : Outport  Port=45
      settings: EnsureOutportIsVirtual=on
  EepMd62ThdRwRtStCshnFldTrgtPos_S_Val_write : Outport  Port=46
      settings: EnsureOutportIsVirtual=on
  EepMd62ThdRwRtStFwdBkwdTrgtPos_S_Val_write : Outport  Port=47
      settings: EnsureOutportIsVirtual=on
  Md62MemReq_Val_write : Outport  Port=48
      settings: EnsureOutportIsVirtual=on
  Md62NotMem_Val_write : Outport  Port=49
      settings: EnsureOutportIsVirtual=on
  wires:
  EepMd62PassStBkReclnTrgtPos_Val_read/1 -> Mux/1
  EepMd62PassStFwdBkwdTrgtPos_Val_read/1 -> Mux/3
  EepMd62SecRwLtStBkReclnTrgtPos_Val_read/1 -> Mux/4
  EepMd62SecRwLtStCushFrntTrgtPos_Val_read/1 -> Mux/5
  EepMd62SecRwLtStFwdBkwdTrgtPos_Val_read/1 -> Mux/6
  EepMd62SecRwLtStLgrstInwdOtwdTrgtPos_Val_read/1 -> Mux/7
  EepMd62SecRwLtStLgrstUpwdDnwdTrgtPos_Val_read/1 -> Mux/8
  EepMd62SecRwRtStBkReclnTrgtPos_Val_read/1 -> Mux/9
  EepMd62SecRwRtStCushFrntTrgtPos_Val_read/1 -> Mux/10
  EepMd62SecRwRtStFwdBkwdTrgtPos_Val_read/1 -> Mux/11
  EepMd62SecRwRtStLgrstInwdOtwdTrgtPos_Val_read/1 -> Mux/12
  EepMd62SecRwRtStLgrstUpwdDnwdTrgtPos_Val_read/1 -> Mux/13
  EepMd62PassStCshnFldTrgtPos_Val_read/1 -> Mux/2
  EepMd62ThdRwLtStFwdBkwdTrgtPos_Val_read/1 -> Mux/16
  EepMd62ThdRwLtStBkReclnTrgtPos_Val_read/1 -> Mux/14
  EepMd62ThdRwRtStBkReclnTrgtPos_Val_read/1 -> Mux/17
  EepMd62ThdRwLtStCshnFldTrgtPos_Val_read/1 -> Mux/15
  EepMd62ThdRwRtStFwdBkwdTrgtPos_Val_read/1 -> Mux/19
  Mux/1 -> Switch/1
  EepMd62ThdRwRtStCshnFldTrgtPos_Val_read/1 -> Mux/18
  Constant/1 -> Unit Delay/1
  Unit Delay1/1 -> Switch/2
  Switch1/1 -> Switch/3
  Unit Delay/1 -> Unit Delay1/1
  MemReq/1 -> Unit Delay3/1, Relational Operator/1
  Constant2/1 -> Relational Operator1/2
  Unit Delay3/1 -> Relational Operator1/1
  Switch/1 -> Unit Delay2/1, Demux/1
  Unit Delay2/1 -> Switch1/3
  Relational Operator/1 -> Logical Operator/1
  Constant1/1 -> Relational Operator/2
  CurrentPosArray/1 -> [CurrentPosArray], Switch1/1
  Relational Operator1/1 -> Logical Operator/2
  Demux/1 -> [PassStBkReclnTrgtPos]
  Demux/2 -> [PassStCshnFldTrgtPos]
  Demux/3 -> [PassStFwdBkwdTrgtPos]
  Demux/4 -> [SecRwLtStBkReclnTrgtPos]
  Demux/5 -> [SecRwLtStCushFrntTrgtPos]
  Demux/6 -> [SecRwLtStFwdBkwdTrgtPos]
  Demux/7 -> [SecRwLtStLgrstInwdOtwdTrgtPos]
  Demux/8 -> [SecRwLtStLgrstUpwdDnwdTrgtPos]
  Demux/9 -> [SecRwRtStBkReclnTrgtPos]
  Demux/10 -> [SecRwRtStCushFrntTrgtPos]
  Demux/11 -> [SecRwRtStFwdBkwdTrgtPos]
  Demux/12 -> [SecRwRtStLgrstInwdOtwdTrgtPos]
  Demux/13 -> [SecRwRtStLgrstUpwdDnwdTrgtPos]
  Demux/14 -> [ThdRwLtStBkReclnTrgtPos]
  Demux/15 -> [ThdRwLtStCshnFldTrgtPos]
  Demux/16 -> [ThdRwLtStFwdBkwdTrgtPos]
  Demux/17 -> [ThdRwRtStBkReclnTrgtPos]
  Demux/18 -> [ThdRwRtStCshnFldTrgtPos]
  Demux/19 -> [ThdRwRtStFwdBkwdTrgtPos]
  Demux1/4 -> Terminator_3/1
  Demux1/11 -> Terminator_10/1
  Demux1/9 -> Terminator_8/1
  Demux1/10 -> Terminator_9/1
  Demux1/16 -> Terminator_13/1
  Demux1/8 -> Terminator_7/1
  Demux1/6 -> Terminator_5/1
  Demux1/5 -> Terminator_4/1
  Demux1/17 -> [ThdRwRtStBkReclnPos]
  Demux1/2 -> [PassStCshnFldPos]
  Demux1/1 -> [PassStBkReclnPos]
  Demux1/15 -> [ThdRwLtStCshnFldPos]
  Demux1/3 -> Terminator_2/1
  Demux1/7 -> Terminator_6/1
  Demux1/18 -> [ThdRwRtStCshnFldPos]
  Demux1/12 -> Terminator_11/1
  Demux1/13 -> Terminator_12/1
  [CurrentPosArray] -> Demux1/1
  Demux1/19 -> Terminator_14/1
  Demux1/14 -> [ThdRwLtStBkReclnPos]
  KeSMSwSeatBkLimitPos_Val/1 -> [SeatBkLimitPos], Add2/1
  Relational Operator3/1 -> Logical Operator2/1
  Relational Operator8/1 -> Logical Operator3/2
  Abs1/1 -> Relational Operator3/1
  Relational Operator7/1 -> Logical Operator5/1
  [ThdRwRtStCshnFldPos] -> Add1/2
  Relational Operator6/1 -> Md62PassStTrgtIsFld_Val_write/1, Logical Operator5/2
  Logical Operator4/1 -> Md62PassStNeedFldOpn_Val_write/1, [PassStNeedFldOpn]
  Relational Operator4/1 -> Logical Operator3/1
  [ThdRwLtStCshnFldPos] -> Add/2
  [ThdRwLtStCshnFldTrgtPos] -> Relational Operator9/1, Add/1
  Add3/1 -> Abs2/1
  KeSMSwSeatBkLimitPosDelt_Val/1 -> [SeatBkLimitPosDelt], Relational Operator8/2, Add2/2
  Logical Operator1/1 -> Md62ThdRwLtStNeedFldOpn_Val_write/1, [ThdLftNeedFldOpn]
  [ThdRwRtStCshnFldTrgtPos] -> Relational Operator10/1, Add1/1
  Relational Operator2/1 -> Logical Operator1/1
  [PassStBkReclnPos] -> Add3/2
  [PassStBkReclnTrgtPos] -> Relational Operator6/1
  ThdRwLtStCshnFldUpwdDnwdMovConfig/1 -> Logical Operator1/2
  ThdRwRtStCshnFldUpwdDnwdMovConfig/1 -> Logical Operator2/2
  Abs/1 -> Relational Operator2/1
  Logical Operator2/1 -> Md62ThdRwRtStNeedFldOpn_Val_write/1, [ThdRghtNeedFldOpn]
  [PassStBkReclnTrgtPos] -> Add3/1
  PA_KeSMSuThrdRwCushFoldPosDelta_Val1/1 -> Relational Operator9/2, Relational Operator2/2
  Abs2/1 -> Relational Operator8/1
  [PassStBkReclnPos] -> Relational Operator4/1
  Add/1 -> Abs/1
  Add1/1 -> Abs1/1
  Add2/1 -> Relational Operator4/2, Relational Operator6/2
  Logical Operator3/1 -> Logical Operator4/1
  PA_KeSMSuThrdRwCushFoldPosDelta_Val2/1 -> Relational Operator10/2, Relational Operator3/2
  [ThdRwRtStBkReclnTrgtPos] -> Mux10/3, Mux10/2, Mux10/1
  Mux8/1 -> Md62ThdRwRtStCshnFldUpwdDnwdTrgtPosCalib_TrgtPosArray_write/1
  Mux9/1 -> Md62SecRwRtStCushFrntTrgtPosCalib_TrgtPosArray_write/1
  [ThdRwLtStCshnFldTrgtPos] -> Md62ThdRwLtStCshnFldUpwdDnwdTrgtPos_Val_write/1, Mux6/1, Mux6/2, Mux6/3
  [ThdRwRtStCshnFldTrgtPos] -> Md62ThdRwRtStCshnFldUpwdDnwdTrgtPos_Val_write/1, Mux8/1, Mux8/2, Mux8/3
  Switch13/1 -> Md62PassStBkReclnTrgtPosCalib_TrgtPosArray_write/1
  Mux5/1 -> Md62ThdRwLtStBkReclnUpwdDnwdTrgtPosCalib_TrgtPosArray_write/1
  Mux10/1 -> Md62ThdRwRtStBkReclnUpwdDnwdTrgtPosCalib_TrgtPosArray_write/1
  [SecRwRtStCushFrntTrgtPos] -> Mux9/3, Mux9/2, Mux9/1
  Mux2/1 -> Md62PassStCshnFldTrgtPosCalib_TrgtPosArray_write/1
  Mux3/1 -> Md62PassStFwdBkwdTrgtPosCalib_TrgtPosArray_write/1
  [ThdRwLtStBkReclnTrgtPos] -> Mux5/3, Mux5/2, Mux5/1
  Mux11/1 -> Md62ThdRwRtStFrwdBkwdPosTrgtPosCalib_TrgtPosArray_write/1
  [PassStCshnFldTrgtPos] -> Mux2/1, Mux2/2, Mux2/3
  Mux6/1 -> Md62ThdRwLtStCshnFldUpwdDnwdTrgtPosCalib_TrgtPosArray_write/1
  [SecRwLtStCushFrntTrgtPos] -> Mux4/1, Mux4/2, Mux4/3
  [PassStBkReclnTrgtPos] -> Md62PassStBkReclnTrgtPos_Val_write/1
  Mux7/1 -> Md62ThdRwLtStFrwdBkwdPosTrgtPosCalib_TrgtPosArray_write/1
  Mux4/1 -> Md62SecRwLtStCushFrntTrgtPosCalib_TrgtPosArray_write/1
  [SecRwLtStFwdBkwdTrgtPos] -> Mux17/3, Mux17/2, Mux17/1
  Mux22/1 -> Switch6/3
  Logical Operator6/1 -> Switch6/2
  [SecRwRtStLgrstInwdOtwdTrgtPos] -> Mux22/3, Mux22/2, Mux22/1
  Mux14/1 -> Switch3/3
  Constant13/1 -> Mux26/1, Mux26/2
  Constant14/1 -> Mux26/3
  [SecRwLtStBkReclnTrgtPos] -> Mux16/1, Mux16/2, Mux16/3
  [ThdLftNeedFldOpn] -> Logical Operator7/1
  [ThdRghtNeedFldOpn] -> Logical Operator7/2
  Constant12/1 -> Mux24/2, Mux24/1
  [PassStNeedFldOpn] -> Logical Operator7/3
  Logical Operator7/1 -> Switch7/2
  Switch5/1 -> Md62SecRwLtStFwdBkwdCalib_TrgtPosArray_write/1
  Switch9/1 -> Md62SecRwRtStFwdBkwdCalib_TrgtPosArray_write/1
  [ThdLftNeedFldOpn] -> Logical Operator6/1
  Mux15/1 -> Switch3/1
  Constant6/1 -> Mux15/3, Mux15/2, Mux15/1
  [ThdRghtNeedFldOpn] -> Logical Operator9/2
  [ThdLftNeedFldOpn] -> Logical Operator9/1
  Mux25/1 -> Switch8/3
  [ThdRghtNeedFldOpn] -> Logical Operator6/2
  Constant10/1 -> Mux20/1, Mux20/2, Mux20/3
  Mux12/1 -> Switch2/1
  [SecRwRtStFwdBkwdTrgtPos] -> Switch9/3
  Mux17/1 -> Switch5/3
  [ThdRghtNeedFldOpn] -> Logical Operator8/2
  Constant5/1 -> Mux12/3, Mux12/2, Mux12/1
  [ThdLftNeedFldOpn] -> Switch2/2
  Constant7/1 -> Mux18/1, Mux18/2
  [ThdLftNeedFldOpn] -> Logical Operator8/1
  [PassStNeedFldOpn] -> Logical Operator6/3
  Mux24/1 -> Switch8/1
  Mux13/1 -> Switch2/3
  Switch6/1 -> Md62SecRwRtStLgrstInwdOtwdTrgtPosCalib_TrgtPosArray_write/1
  [SecRwRtStLgrstUpwdDnwdTrgtPos] -> Mux23/3, Mux23/2, Mux23/1
  Mux21/1 -> Switch7/1
  Constant9/1 -> Mux19/3
  Switch3/1 -> Md62SecRwLtStLgrstUpwdDnwdTrgtPosCalib_TrgtPosArray_write/1
  [SecRwRtStBkReclnTrgtPos] -> Mux25/1, Mux25/2, Mux25/3
  Constant11/1 -> Mux21/3, Mux21/2, Mux21/1
  Mux26/1 -> Switch9/1
  [ThdLftNeedFldOpn] -> Switch3/2
  [SecRwLtStLgrstInwdOtwdTrgtPos] -> Mux13/1, Mux13/2, Mux13/3
  [SecRwLtStLgrstUpwdDnwdTrgtPos] -> Mux14/3, Mux14/2, Mux14/1
  Switch4/1 -> Md62SecRwLtStBkReclnTrgtPosCalib_TrgtPosArray_write/1
  Mux16/1 -> Switch4/3
  Mux20/1 -> Switch6/1
  Constant8/1 -> Mux19/2, Mux19/1
  Switch7/1 -> Md62SecRwRtStLgrstUpwdDnwdTrgtPosCalib_TrgtPosArray_write/1
  Mux19/1 -> Switch5/1
  Switch8/1 -> Md62SecRwRtStBkReclnTrgtPosCalib_TrgtPosArray_write/1
  Mux23/1 -> Switch7/3
  Mux18/1 -> Switch4/1
  Switch2/1 -> Md62SecRwLtStLgrstInwdOtwdTrgtPosCalib_TrgtPosArray_write/1
  Relational Operator9/1 -> Md62ThdRwLtStTrgtIsFld_Val_write/1
  Relational Operator10/1 -> Md62ThdRwRtStTrgtIsFld_Val_write/1
  Constant18/1 -> Switch11/1
  Relational Operator12/1 -> Switch11/2
  Constant16/1 -> Switch10/1
  [ThdRwLtStCshnFldTrgtPos] -> Add4/2
  Add4/1 -> Relational Operator11/1
  Relational Operator11/1 -> Switch10/2
  PA_KeSMSuThrdRwCushFoldPosDelta_Val3/1 -> Relational Operator11/2
  [ThdRwLtStFwdBkwdTrgtPos] -> Switch10/3
  Switch11/1 -> Mux11/1, Mux11/2, Mux11/3
  Switch10/1 -> Mux7/1, Mux7/3, Mux7/2
  [ThdRwRtStFwdBkwdTrgtPos] -> Switch11/3
  [ThdRwLtStCshnFldPos] -> Add4/1
  Add5/1 -> Relational Operator12/1
  [ThdRwRtStCshnFldPos] -> Add5/1
  [ThdRwRtStCshnFldTrgtPos] -> Add5/2
  PA_KeSMSuThrdRwCushFoldPosDelta_Val4/1 -> Relational Operator12/2
  [SeatBkLimitPos] -> Add6/1
  Relational Operator13/1 -> Logical Operator10/1
  Relational Operator14/1 -> Logical Operator10/2
  [PassStBkReclnPos] -> Relational Operator13/1
  [PassStFwdBkwdTrgtPos] -> Switch12/3
  PA_KeSMSwAcsMd30PassStFrwdBkwdPos1_Val/1 -> Switch12/1
  [PassStBkReclnPos] -> Relational Operator14/1
  [SeatBkLimitPosDelt] -> Add6/2
  Add6/1 -> Relational Operator13/2
  PA_KeSMSuFirstRwStBackPosDelta_Val2/1 -> Relational Operator14/2
  Switch15/1 -> Mux3/2, Mux3/1, Mux3/3
  Mux28/1 -> Switch13/3
  PA_KeSMSwAcsMd30PassStBkReclnUpwdDnwdPos1Max_Val1/1 -> Mux27/2
  Relational Operator15/1 -> Logical Operator11/1
  Logical Operator11/1 -> Switch13/2
  PA_KeSMSwAcsMd30PassStBkReclnUpwdDnwdPos1Min_Val1/1 -> Mux27/3
  Mux27/1 -> Switch13/1
  PA_KeSMSwAcsMd30PassStBkReclnUpwdDnwdPos1_Val1/1 -> Mux27/1
  [PassStBkReclnTrgtPos] -> Mux28/3, Mux28/1, Mux28/2
  [PassStCshnFldPos] -> Relational Operator15/1
  [PassStNeedFld] -> Logical Operator11/2
  PA_KeSMSwAcsMd30PassStFldUpwdDnwdPos1_Val/1 -> Relational Operator15/2
  [PassStBkReclnTrgtPos] -> EepMd62PassStBkReclnTrgtPos_S_Val_write/1
  [PassStCshnFldTrgtPos] -> EepMd62PassStCshnFldTrgtPos_S_Val_write/1
  [PassStFwdBkwdTrgtPos] -> EepMd62PassStFwdBkwdTrgtPos_S_Val_write/1
  [ThdRwRtStFwdBkwdTrgtPos] -> EepMd62ThdRwRtStFwdBkwdTrgtPos_S_Val_write/1
  [ThdRwRtStCshnFldTrgtPos] -> EepMd62ThdRwRtStCshnFldTrgtPos_S_Val_write/1
  [ThdRwRtStBkReclnTrgtPos] -> EepMd62ThdRwRtStBkReclnTrgtPos_S_Val_write/1
  [ThdRwLtStFwdBkwdTrgtPos] -> EepMd62ThdRwLtStFwdBkwdTrgtPos_S_Val_write/1
  [ThdRwLtStCshnFldTrgtPos] -> EepMd62ThdRwLtStCshnFldTrgtPos_S_Val_write/1
  [ThdRwLtStBkReclnTrgtPos] -> EepMd62ThdRwLtStBkReclnTrgtPos_S_Val_write/1
  [SecRwRtStLgrstUpwdDnwdTrgtPos] -> EepMd62SecRwRtStLgrstUpwdDnwdTrgtPos_S_Val_write/1
  [SecRwRtStLgrstInwdOtwdTrgtPos] -> EepMd62SecRwRtStLgrstInwdOtwdTrgtPos_S_Val_write/1
  [SecRwRtStFwdBkwdTrgtPos] -> EepMd62SecRwRtStFwdBkwdTrgtPos_S_Val_write/1
  [SecRwRtStCushFrntTrgtPos] -> EepMd62SecRwRtStCushFrntTrgtPos_S_Val_write/1
  [SecRwRtStBkReclnTrgtPos] -> EepMd62SecRwRtStBkReclnTrgtPos_S_Val_write/1
  [SecRwLtStLgrstUpwdDnwdTrgtPos] -> EepMd62SecRwLtStLgrstUpwdDnwdTrgtPos_S_Val_write/1
  [SecRwLtStLgrstInwdOtwdTrgtPos] -> EepMd62SecRwLtStLgrstInwdOtwdTrgtPos_S_Val_write/1
  [SecRwLtStFwdBkwdTrgtPos] -> EepMd62SecRwLtStFwdBkwdTrgtPos_S_Val_write/1
  [SecRwLtStCushFrntTrgtPos] -> EepMd62SecRwLtStCushFrntTrgtPos_S_Val_write/1
  [SecRwLtStBkReclnTrgtPos] -> EepMd62SecRwLtStBkReclnTrgtPos_S_Val_write/1
  Logical Operator5/1 -> Logical Operator4/2, [PassStNeedFld]
  Add8/1 -> Relational Operator7/1
  [PassStBkReclnPos] -> Add8/1
  PA_KeSMSuFirstRwStBackPosDelta_Val1/1 -> Relational Operator7/2
  [PassStBkReclnTrgtPos] -> Add8/2
  [PassStBkReclnTrgtPos] -> Relational Operator16/1
  Constant21/1 -> Relational Operator16/2
  Relational Operator16/1 -> Md62NotMem_Val_write/1
  [PassStNeedFldOpn] -> Logical Operator12/2
  Logical Operator12/1 -> Switch12/2
  Logical Operator10/1 -> Logical Operator12/1
  Constant23/1 -> Relational Operator18/2
  IfVeSMSuSecRwLtStBkReclnUpwdDnwdPos/1 -> Relational Operator18/1
  [ThdLftNeedFldOpn] -> Switch4/2
  [ThdLftNeedFldOpn] -> Switch5/2
  Constant22/1 -> Relational Operator17/2
  IfVeSMSuSecRwLtStFrwdBkwdPos/1 -> Relational Operator17/1
  Constant24/1 -> Relational Operator19/2
  IfVeSMSuSecRwRtStBkReclnUpwdDnwdPos/1 -> Relational Operator19/1
  Logical Operator8/1 -> Switch8/2
  Constant25/1 -> Relational Operator20/2
  IfVeSMSuSecRwRtStFrwdBkwdPos/1 -> Relational Operator20/1
  Logical Operator9/1 -> Switch9/2
  Constant26/1 -> Mux18/3
  Relational Operator17/1 -> Terminator_15/1
  Relational Operator18/1 -> Terminator_16/1
  Relational Operator19/1 -> Terminator_17/1
  Relational Operator20/1 -> Terminator_18/1
  PA_KeSMSuFirstRwStFwdBkwdPosDelta_Val/1 -> Terminator_19/1
  PA_KeSMSwAcsMd30PassStFrwdBkwdPos1Max_Val/1 -> Terminator_21/1
  PA_KeSMSuThrdRwCushFoldPosDelta_Val/1 -> Terminator_20/1
  PA_KeSMSuFirstRwStCushFoldPosDelta_Val/1 -> Terminator_1/1
  PA_KeSMSwAcsMd30PassStFrwdBkwdPos1Min_Val/1 -> Terminator_22/1
  Constant3/1 -> Mux24/3
  modestate32_Val_read/1 -> 32BitSelector2/1
  32BitSelector2/1 -> Switch14/2
  Constant4/1 -> Switch14/1
  Logical Operator/1 -> Switch14/3
  Switch14/1 -> Switch1/2, Md62MemReq_Val_write/1
  IfVeSMSuPassStBkReclnUpwdDnwdPosV/1 -> Switch15/2
  Switch12/1 -> Switch15/3
  Constant15/1 -> Switch15/1
